simulink model "WaterTankProcess_model"  (R2016a)
settings: Solver=ode4  StartTime=0.0  StopTime=SIM_TIME  FixedStep=STEP_SIZE  RelTol=1e-3
values from neighbouring files (symbols this model uses):
  At = 0.785    [TwoTankSystem.m]
  Av0 = 0.0122    [TwoTankSystem.m]
  Av1 = 1.05*Av0    (= 0.01281)    [TwoTankSystem.m]
  C0 = 0.056    [TwoTankSystem.m]
  Dv = 2.66    [TwoTankSystem.m]
  ka = 0.004    [TwoTankSystem.m]
  kh = 2    [TwoTankSystem.m]
  kt = 0.1    [TwoTankSystem.m]
  Tc = 400    [TwoTankSystem.m]
  Tc0 = 30    [TwoTankSystem.m]
  Tc1 = 1.2*Tc0    (= 36)    [TwoTankSystem.m]
  Tv = 700    [TwoTankSystem.m]
  Tw = 100    [TwoTankSystem.m]
  Tw0 = 60    [TwoTankSystem.m]
  Tw1 = 1.1*Tw0    (= 66)    [TwoTankSystem.m]
  uc0 = 5    [TwoTankSystem.m]
  uc1 = 0.9*uc0    (= 4.5)    [TwoTankSystem.m]
  uw0 = 5    [TwoTankSystem.m]
  uw1 = 1.1*uw0    (= 5.5)    [TwoTankSystem.m]
  x0 = xFinal'    [TwoTankSystem.m]
undefined symbols (not defined in the file or in its folder): T1, T2
settings Model: Creator=roga  LastModifiedBy=Roberto
settings DataIOCC: LimitDataPoints=on  SaveFinalState=on  SaveFormat=Array
settings DebuggingCC: UnderspecifiedInitializationDetection=Classic  MergeDetectMultiDrivingBlocksExec=none  SolverPrmCheckMsg=warning  StateNameClashWarn=warning
settings HardwareCC: ProdBitPerPointer=32  ProdLargestAtomicFloat=None  ProdIntDivRoundTo=Undefined  ProdEndianess=Unspecified  ProdWordSize=32  ProdHWDeviceType=32-bit Generic
settings ModelReferenceCC: PropagateSignalLabelsOutOfModel=off
settings ConfigComp: CovModelRefEnable=Off

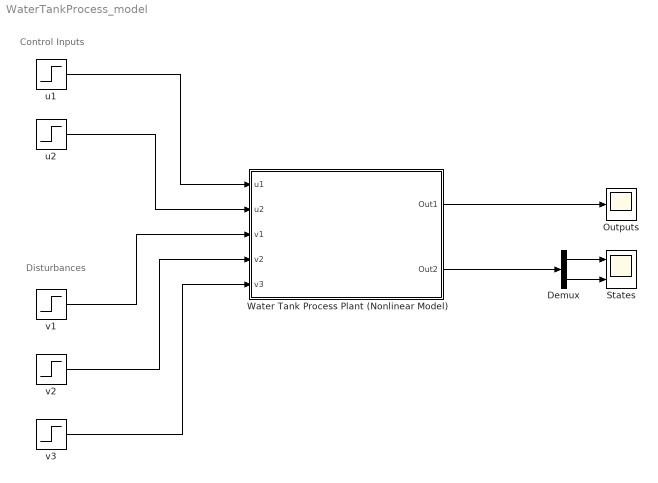
== system WaterTankProcess_model ==
  note: Disturbances
  note: Control Inputs
  Demux : Demux  Outputs=2
  Outputs : Scope
  States : Scope  NumInputPorts=2
  Water Tank Process Plant (Nonlinear Model) : Subsystem
      mask Display:
      | port_label('output',1,'y','texmode','on')
      | port_label('output',2,'x','texmode','on')
      | port_label('input',1,'u_1','texmode','on')
      | port_label('input',2,'u_2','texmode','on')
      | port_label('input',3,'A_v','texmode','on')
      | port_label('input',4,'T_w','texmode','on')
      | port_label('input',5,'T_c','texmode','on')
  u1 : Step  Time=Tw  Before=uw0  After=uw1  SampleTime=0
  u2 : Step  Time=Tc  Before=uc0  After=uc1  SampleTime=0
  v1 : Step  Time=Tv  Before=Av0  After=Av1  SampleTime=0
  v2 : Step  Time=T1  Before=Tw0  After=Tw1  SampleTime=0
  v3 : Step  Time=T2  Before=Tc0  After=Tc1  SampleTime=0
  wires:
  Demux/1 -> States/1
  Demux/2 -> States/2
  u1/1 -> Water Tank Process Plant (Nonlinear Model)/1(u1)
  u2/1 -> Water Tank Process Plant (Nonlinear Model)/2(u2)
  v1/1 -> Water Tank Process Plant (Nonlinear Model)/3(v1)
  v2/1 -> Water Tank Process Plant (Nonlinear Model)/4(v2)
  v3/1 -> Water Tank Process Plant (Nonlinear Model)/5(v3)
  Water Tank Process Plant (Nonlinear Model)/1(Out1) -> Outputs/1
  Water Tank Process Plant (Nonlinear Model)/2(Out2) -> Demux/1

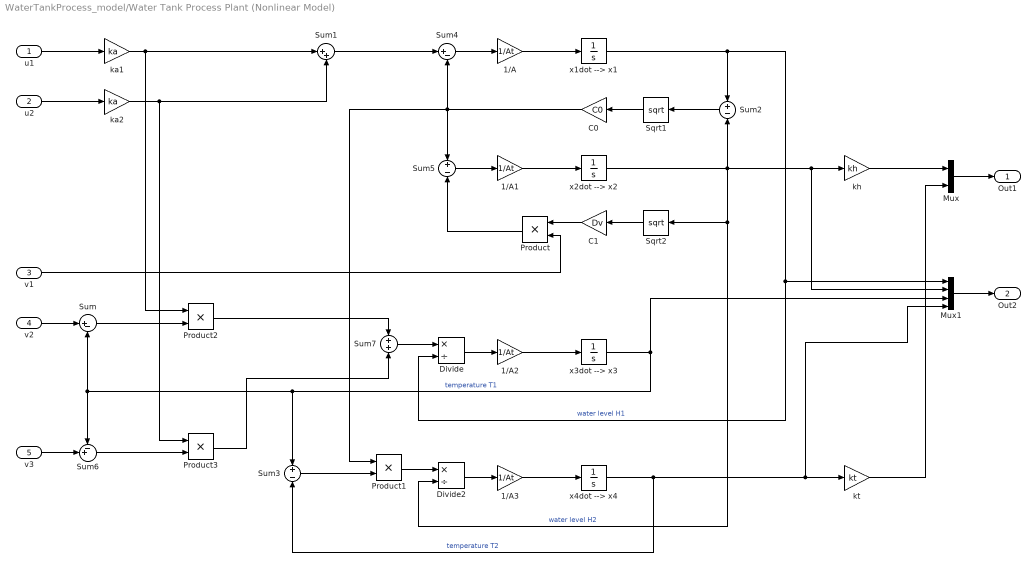
== system WaterTankProcess_model/Water Tank Process Plant (Nonlinear Model) ==
  u1 : Inport
  u2 : Inport  Port=2
  v1 : Inport  Port=3
  v2 : Inport  Port=4
  v3 : Inport  Port=5
  1/A{,1..3} (4 alike) : Gain  Gain=1/At
  C0 : Gain  Gain=C0
  C1 : Gain  Gain=Dv
  Divide : Product  Inputs=*/
  Divide2 : Product  Inputs=*/
  Mux : Mux  Inputs=2
  Mux1 : Mux
  Product{,1..3} (4 alike) : Product
  Sqrt1 : Sqrt  SaturateOnIntegerOverflow=on
  Sqrt2 : Sqrt  SaturateOnIntegerOverflow=on
  Sum : Sum  Inputs=|+-
  Sum1 : Sum  Inputs=|++
  Sum2 : Sum  Inputs=+-
  Sum3 : Sum  Inputs=+-
  Sum4 : Sum  Inputs=|+-
  Sum5 : Sum  Inputs=+-
  Sum6 : Sum  Inputs=-+|
  Sum7 : Sum
  ka1 : Gain  Gain=ka
  ka2 : Gain  Gain=ka
  kh : Gain  Gain=kh
  kt : Gain  Gain=kt
  x1dot --> x1 : Integrator  InitialCondition=x0(1)  LimitOutput=on  LowerSaturationLimit=0
  x2dot --> x2 : Integrator  InitialCondition=x0(2)  LimitOutput=on  LowerSaturationLimit=0
  x3dot --> x3 : Integrator  InitialCondition=x0(3)
  x4dot --> x4 : Integrator  InitialCondition=x0(4)
  Out1 : Outport
  Out2 : Outport  Port=2
  wires:
  Product1/1 -> Divide2/1
  u2/1 -> ka2/1
  Divide/1 -> 1/A2/1
  Sum6/1 -> Product3/2
  v2/1 -> Sum/1
  1/A1/1 -> x2dot --> x2/1
  Sum5/1 -> 1/A1/1
  Product/1 -> Sum5/2
  x1dot --> x1/1 -> Sum2/1, Mux1/1, Divide/2  "water level H1"
  Sum/1 -> Product2/2
  C1/1 -> Product/1
  Sum3/1 -> Product1/2
  Sqrt2/1 -> C1/1
  1/A2/1 -> x3dot --> x3/1
  u1/1 -> ka1/1
  v1/1 -> Product/2
  kh/1 -> Mux/1
  x4dot --> x4/1 -> Mux1/4, kt/1, Sum3/2  "temperature T2"
  C0/1 -> Sum4/2, Product1/1, Sum5/1
  1/A3/1 -> x4dot --> x4/1
  x2dot --> x2/1 -> Mux1/2, kh/1, Divide2/2, Sqrt2/1, Sum2/2  "water level H2"
  Divide2/1 -> 1/A3/1
  Sum7/1 -> Divide/1
  v3/1 -> Sum6/2
  Product2/1 -> Sum7/1
  ka1/1 -> Product2/1, Sum1/1
  Product3/1 -> Sum7/2
  Mux/1 -> Out1/1
  ka2/1 -> Product3/1, Sum1/2
  kt/1 -> Mux/2
  x3dot --> x3/1 -> Sum3/1, Sum6/1, Sum/2, Mux1/3  "temperature T1"
  1/A/1 -> x1dot --> x1/1
  Sum1/1 -> Sum4/1
  Mux1/1 -> Out2/1
  Sqrt1/1 -> C0/1
  Sum4/1 -> 1/A/1
  Sum2/1 -> Sqrt1/1
